simulink model "compare_linear_vs_non_linear_simulation"  (R2020a)
settings: Solver=ode4  StartTime=0.0  StopTime=80  FixedStep=0.01  RelTol=1e-3
InitFcn:
  | linearize_script;
undefined symbols (not defined in the file): Ac, Bc, th_op, Vmp_op, Vmy_op, w_th_op, w_yw_op, yw_op
libraries: realtime_pacer_lib x1
settings Model: Creator=engen  LastModifiedBy=engen

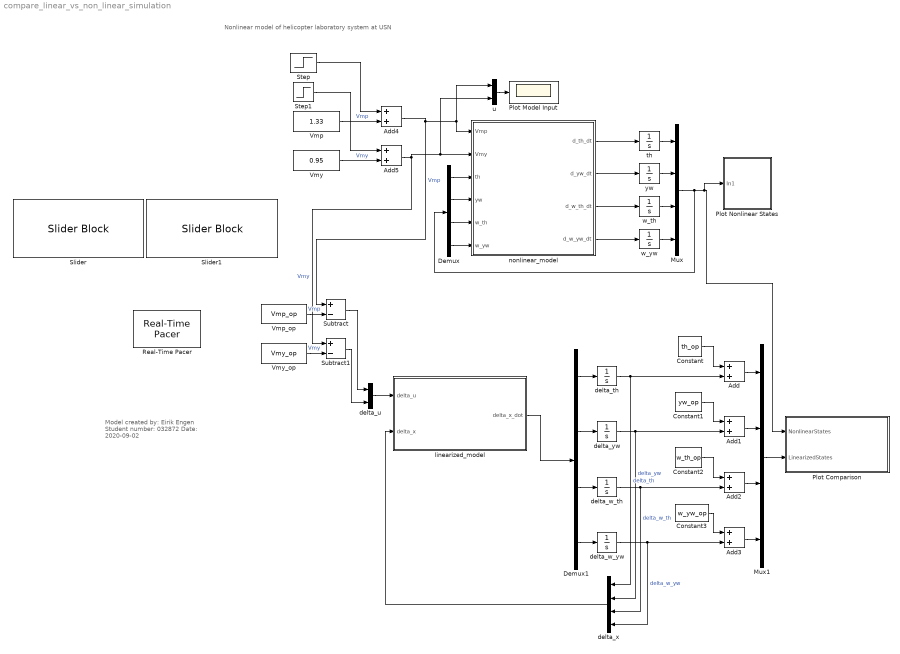
== system compare_linear_vs_non_linear_simulation ==
  note: Model created by: Eirik Engen
      | Student number: 032872
      | Date: 2020-09-02
  note: Nonlinear model of helicopter laboratory system at USN
  Add{,1..5} (6 alike) : Sum
  Constant : Constant  Value=th_op
  Constant1 : Constant  Value=yw_op
  Constant2 : Constant  Value=w_th_op
  Constant3 : Constant  Value=w_yw_op
  Demux : Demux
  Demux1 : Demux
  Mux : Mux
  Mux1 : Mux
  Plot Comparison : Subsystem  TreatAsAtomicUnit=on
  Plot Model Input : Scope
  Plot Nonlinear States : Subsystem
  Real-Time Pacer : realtime_pacer_lib/Real-Time Pacer  simTimePerRealTime=10
  Slider : SliderBlock  ScaleMax=1.5
  Slider1 : SliderBlock  ScaleMax=1.5
  Step : Step  Time=20  After=0.02  SampleTime=0
  Step1 : Step  Time=40  After=0.01  SampleTime=0
  Subtract : Sum  Inputs=+-
  Subtract1 : Sum  Inputs=+-
  Vmp : Constant  Value=1.33  SampleTime=-1
  Vmp_op : Constant  Value=Vmp_op  SampleTime=-1
  Vmy : Constant  Value=0.95  SampleTime=-1
  Vmy_op : Constant  Value=Vmy_op  SampleTime=-1
  delta_th : Integrator  ContinuousStateAttributes='w_yw'
  delta_u : Mux  Inputs=2
  delta_w_th : Integrator
  delta_w_yw : Integrator
  delta_x : Mux
  delta_yw : Integrator
  linearized_model : MATLAB Function  TreatAsAtomicUnit=on
  nonlinear_model : MATLAB Function  TreatAsAtomicUnit=on
  th : Integrator  InitialCondition=-10*pi/180  LimitOutput=on  UpperSaturationLimit=45*pi/180  LowerSaturationLimit=-45*pi/180  ContinuousStateAttributes='th'
  u : Mux  Inputs=2
  w_th : Integrator  ContinuousStateAttributes='w_th'
  w_yw : Integrator  ContinuousStateAttributes='w_yw'
  yw : Integrator  InitialCondition=pi/2  LimitOutput=on  UpperSaturationLimit=180*pi/180  LowerSaturationLimit=0  ContinuousStateAttributes='yw'
  wires:
  Add4/1 -> Subtract/1, nonlinear_model/1(Vmp), u/1  "Vmp"
  Add5/1 -> u/2, nonlinear_model/2(Vmy), Subtract1/1  "Vmy"
  nonlinear_model/1(d_th_dt) -> th/1
  nonlinear_model/2(d_yw_dt) -> yw/1
  nonlinear_model/3(d_w_th_dt) -> w_th/1
  nonlinear_model/4(d_w_yw_dt) -> w_yw/1
  th/1 -> Mux/1
  yw/1 -> Mux/2
  w_th/1 -> Mux/3
  w_yw/1 -> Mux/4
  Mux/1 -> Plot Comparison/1(NonlinearStates), Plot Nonlinear States/1(In1), Demux/1
  Demux/1 -> nonlinear_model/3(th)
  Demux/2 -> nonlinear_model/4(yw)
  Demux/3 -> nonlinear_model/5(w_th)
  Demux/4 -> nonlinear_model/6(w_yw)
  u/1 -> Plot Model Input/1
  delta_u/1 -> linearized_model/1(delta_u)
  Vmp_op/1 -> Subtract/2  "Vmp"
  Subtract/1 -> delta_u/1
  Vmy_op/1 -> Subtract1/2  "Vmy"
  Subtract1/1 -> delta_u/2
  linearized_model/1(delta_x_dot) -> Demux1/1
  Demux1/1 -> delta_th/1
  Demux1/2 -> delta_yw/1
  Demux1/3 -> delta_w_th/1
  Demux1/4 -> delta_w_yw/1
  Constant/1 -> Add/1
  Constant1/1 -> Add1/1
  Constant2/1 -> Add2/1
  Constant3/1 -> Add3/1
  Add/1 -> Mux1/1
  Add1/1 -> Mux1/2
  Add2/1 -> Mux1/3
  Add3/1 -> Mux1/4
  Mux1/1 -> Plot Comparison/2(LinearizedStates)
  delta_th/1 -> delta_x/1, Add/2  "delta_th"
  delta_yw/1 -> delta_x/2, Add1/2  "delta_yw"
  delta_w_th/1 -> delta_x/3, Add2/2  "delta_w_th"
  delta_w_yw/1 -> delta_x/4, Add3/2  "delta_w_yw"
  delta_x/1 -> linearized_model/2(delta_x)
  Vmp/1 -> Add4/2  "Vmp"
  Vmy/1 -> Add5/2  "Vmy"
  Step/1 -> Add4/1
  Step1/1 -> Add5/1

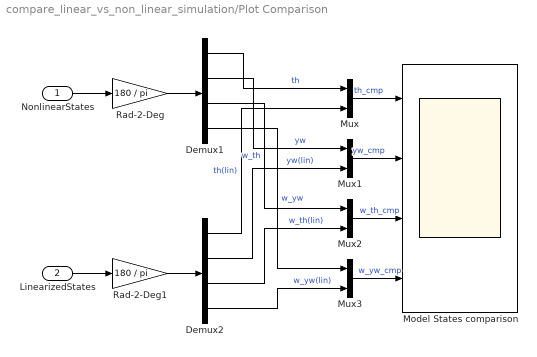
== system compare_linear_vs_non_linear_simulation/Plot Comparison ==
  NonlinearStates : Inport
  LinearizedStates : Inport  Port=2
  Demux1 : Demux
  Demux2 : Demux
  Model States comparison : Scope  NumInputPorts=4
  Mux{,1..3} (4 alike) : Mux  Inputs=2
  Rad-2-Deg : Gain  Gain=180 / pi
  Rad-2-Deg1 : Gain  Gain=180 / pi
  wires:
  NonlinearStates/1 -> Rad-2-Deg/1
  Rad-2-Deg/1 -> Demux1/1
  LinearizedStates/1 -> Rad-2-Deg1/1
  Rad-2-Deg1/1 -> Demux2/1
  Mux/1 -> Model States comparison/1  "th_cmp"
  Mux1/1 -> Model States comparison/2  "yw_cmp"
  Mux2/1 -> Model States comparison/3  "w_th_cmp"
  Mux3/1 -> Model States comparison/4  "w_yw_cmp"
  Demux2/4 -> Mux3/2  "w_yw(lin)"
  Demux1/4 -> Mux3/1  "w_yw"
  Demux2/3 -> Mux2/2  "w_th(lin)"
  Demux1/3 -> Mux2/1  "w_th"
  Demux2/2 -> Mux1/2  "yw(lin)"
  Demux1/2 -> Mux1/1  "yw"
  Demux2/1 -> Mux/2  "th(lin)"
  Demux1/1 -> Mux/1  "th"

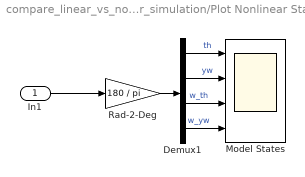
== system compare_linear_vs_non_linear_simulation/Plot Nonlinear States ==
  In1 : Inport
  Demux1 : Demux
  Model States : Scope  NumInputPorts=4
  Rad-2-Deg : Gain  Gain=180 / pi
  wires:
  In1/1 -> Rad-2-Deg/1
  Demux1/2 -> Model States/2  "yw"
  Demux1/3 -> Model States/3  "w_th"
  Demux1/1 -> Model States/1  "th"
  Demux1/4 -> Model States/4  "w_yw"
  Rad-2-Deg/1 -> Demux1/1

== matlab function compare_linear_vs_non_linear_simulation/linearized_model ==
  data: delta_u input; delta_x_dot output; delta_x input; Ac parameter; Bc parameter
% Simulink linearized model of USN helicopter
% Author: Eirik Engen
% Date: 2020-09-02

function delta_x_dot  = linearized_model(delta_u, delta_x, Ac, Bc)

delta_x_dot = Ac*delta_x + Bc*delta_u;

== matlab function compare_linear_vs_non_linear_simulation/nonlinear_model ==
  data: Vmp input; d_th_dt output; Vmy input; th input; yw input; w_th input; w_yw input; d_yw_dt output; d_w_th_dt output; d_w_yw_dt output
% Simulink nonlinear model of USN helicopter
% Author: Eirik Engen
% Date: 2020-09-02

function [d_th_dt, d_yw_dt, d_w_th_dt, d_w_yw_dt] = non_linear_model(Vmp, Vmy, th, yw, w_th, w_yw)          %#ok<INUSL>
% function inputs
% Vmp : Model input - Voltage input to Pitch motor/rotor [V]
% Vmy : Model input - Voltage input to Yaw motor/rotor [V]
% th  : Model state - Pitch angle, theta [radians]
% yw  : Model state - Yaw angle, psi [radians]
% w_th: Model state - Pitch angular velocity, omega_theta [radians / s]
% w_yw: Model state - Yaw angular velocity, omega_psi [radians / s]

% System parameters
l_cm   = 0.015;   % [m] - Distance between the pivot point and the center of mass of the helicopter.
m_heli = 0.479;   % [kg] - Total moving mass of the helicopter
J_eq_p = 0.0172;  % [kg-m^2] - Moment of inertia about pitch axis
J_eq_y = 0.0210;  % [kg-m^2] - Moment of inertia about yaw axis
g      = 9.81;    % [m/s^2] - Acceleration due to gravity on planet earth

Kpp    = 0.0556;  % [Nm/V] - Torque constant on pitch axis from pitch motor
Kyy    = 0.21084; % [Nm/V] - Torque constant on yaw axis from yaw motor
Kpy    = 0.005;   % [Nm/V] - Torque constant on pitch axis from yaw motor
Kyp    = 0.15;    % [Nm/V] - Torque constant on yaw axis from pitch motor
Bp     = 0.01;    % [N/V]  - Damping friction factor about pitch axis
By     = 0.08;    % [N/V]  - Damping friction factor about yaw axis

% Differential equations
d_th_dt = w_th;
d_yw_dt = w_yw;
d_w_th_dt = (Kpp*Vmp - ...
    Kpy*Vmy - ...
    Bp*w_th - ...
    m_heli*l_cm^2*w_yw^2*sin(th)*cos(th) - ...
    m_heli*g*l_cm*cos(th)) / ...
    (J_eq_p+m_heli*l_cm^2);
d_w_yw_dt = (Kyp*Vmp - ...
    Kyy*Vmy - ...
    By*w_yw + ...
    2*m_heli*l_cm^2*w_th*w_yw*sin(th)*cos(th)) / ...
    (J_eq_y+m_heli*l_cm^2*cos(th)^2);
